simulink model "sampleModel2068_2_sub_sub"  (R2023a)
settings: Solver=VariableStepAuto  StartTime=0.0  StopTime=10.0  RelTol=1e-3
libraries: hdlsllib x2, simulink x2
settings Model: Creator=user1  LastModifiedBy=user1

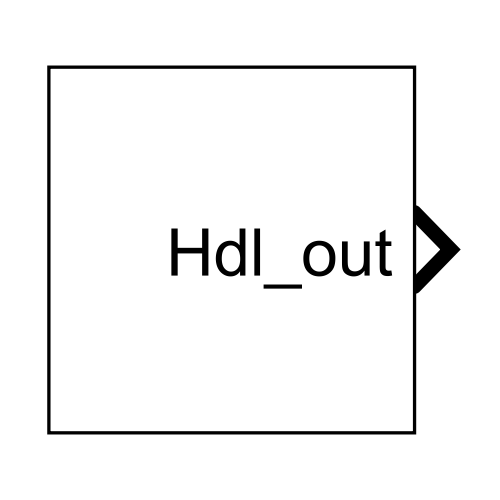
[thumbnail: Simulink's stored preview of the top-level diagram]
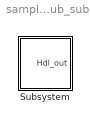
== system sampleModel2068_2_sub_sub ==
  Subsystem : Subsystem

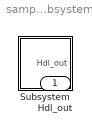
== system sampleModel2068_2_sub_sub/Subsystem ==
  Subsystem : Subsystem
  Hdl_out : Outport  OutDataTypeStr=uint8

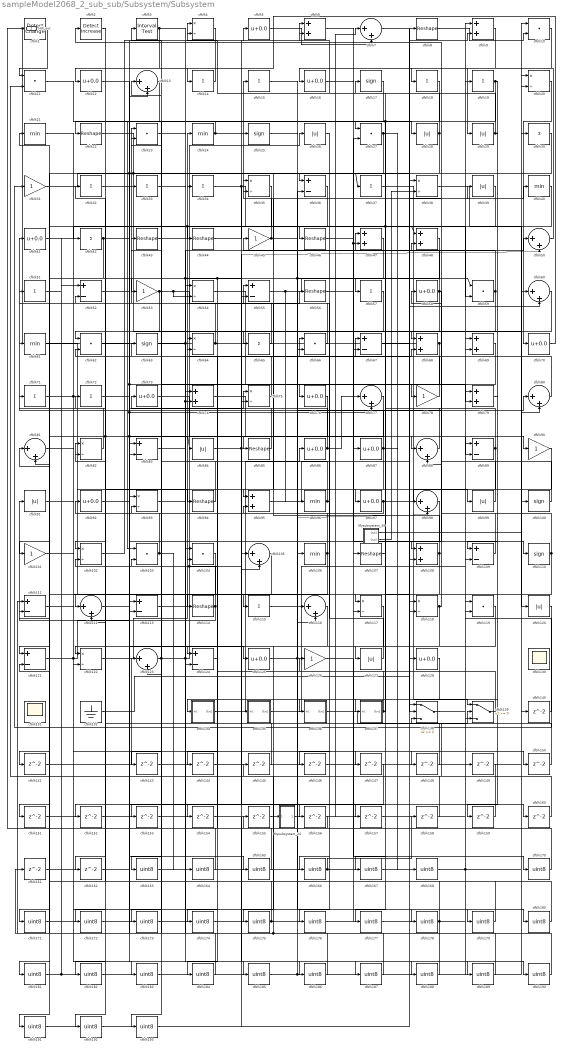
== system sampleModel2068_2_sub_sub/Subsystem/Subsystem ==
  Mysubsystem_24 : Subsystem  TreatAsAtomicUnit=on  RTWFcnName=Mysubsystem_24
      settings: RTWFcnNameOpts=User specified  RTWFileNameOpts=Use function name
  Mysubsystem_45 : Subsystem  TreatAsAtomicUnit=on  RTWFcnName=Mysubsystem_45
      settings: RTWFcnNameOpts=User specified  RTWFileNameOpts=Use function name
  cfblk1 : simulink/Logic and Bit Operations/Detect Change  vinit=0  OutDataTypeStr=uint8
      settings: LibrarySourceBlock=|
      | hdlsllib/Logic and Bit
      | Operations/Detect
      | Change
  cfblk{10..11,23,27,59,62,66,103..104,119} (10 alike) : DotProduct  OutDataTypeStr=uint8
  cfblk{17,25,63,100,110} (5 alike) : Signum
  cfblk{31,45,53,78,90,101,126} (7 alike) : Gain  OutDataTypeStr=uint8
  cfblk{4,20,35,38,54,64,75,82,93,102,117..118,122} (13 alike) : Product  Inputs=*/  OutDataTypeStr=uint8  RndMeth=Zero  SaturateOnIntegerOverflow=on
  cfblk{7,13,50,60,77,80..81,88,98,105,112,116,123} (13 alike) : Sum  Inputs=|++  OutDataTypeStr=uint8
  cfblk{21,24,40,61,96,106} (6 alike) : MinMax  OutDataTypeStr=uint8
  cfblk{8,22,43..44,46,56,85,94,107,114} (10 alike) : Reshape
  cfblk{6,9,47..48,68..69,74,79,95,108} (10 alike) : Sum  OutDataTypeStr=uint8
  cfblk{36,52,55,67,83,89,109,111,113,121,124} (11 alike) : Sum  Inputs=+-  OutDataTypeStr=uint8
  cfblk{14..15,18..19,30,32..34,37,42,51,57,65,71..72,115} (16 alike) : Sum  Inputs=+  OutDataTypeStr=uint8
  cfblk{5,12,16,41,58,70,73,76,86..87,92,97,125,128} (14 alike) : Bias  Bias=0.0  SaturateOnIntegerOverflow=off
  cfblk{26,28..29,39,84,91,99,120,127} (9 alike) : Abs  OutDataTypeStr=uint8  SaturateOnIntegerOverflow=off
  cfblk130 : Scope
      settings: Floating=on
  cfblk131 : Scope
      settings: Floating=on
  cfblk132 : Ground
  cfblk134 : Subsystem
      settings: LibrarySourceBlock=|
      | hdlsllib/Ports &
      | Subsystems/Subsystem
  cfblk135 : Subsystem
      settings: LibrarySourceBlock=|
      | hdlsllib/Ports &
      | Subsystems/Subsystem
  cfblk136 : Subsystem
      settings: LibrarySourceBlock=|
      | hdlsllib/Ports &
      | Subsystems/Subsystem
  cfblk137 : Subsystem
      settings: LibrarySourceBlock=|
      | hdlsllib/Ports &
      | Subsystems/Subsystem
  cfblk138 : Switch  OutDataTypeStr=uint8  SaturateOnIntegerOverflow=off  InputSameDT=off
  cfblk139 : Switch  OutDataTypeStr=uint8  SaturateOnIntegerOverflow=off  InputSameDT=off
  cfblk{140..141,143..162} (22 alike) : Delay  SampleTime=1
  cfblk{163..168,170..193} (30 alike) : DataTypeConversion  OutDataTypeStr=uint8  SaturateOnIntegerOverflow=off  RndMeth=Floor
  cfblk2 : simulink/Logic and Bit Operations/Detect Increase  vinit=0.0  OutDataTypeStr=uint8
      settings: LibrarySourceBlock=|
      | hdlsllib/Logic and Bit
      | Operations/Detect
      | Increase
  cfblk3 : hdlsllib/Logic and Bit Operations/Interval Test  IntervalClosedRight=on  uplimit=0.5  IntervalClosedLeft=on  lowlimit=-0.5  OutDataTypeStr=uint8
  Hdl_out : Outport  OutDataTypeStr=uint8
  wires:
  Mysubsystem_45/2(Out2) -> cfblk38/2
  Mysubsystem_45/1(Out1) -> cfblk10/1
  Mysubsystem_24/1(Out1) -> cfblk7/1
  cfblk83/1 -> Mysubsystem_24/1(In1)
  cfblk193/1 -> cfblk105/2
  cfblk60/1 -> cfblk193/1
  cfblk192/1 -> cfblk105/1
  cfblk147/1 -> cfblk192/1
  cfblk191/1 -> cfblk8/1
  cfblk105/1 -> cfblk191/1
  cfblk190/1 -> cfblk93/2
  cfblk154/1 -> cfblk190/1
  cfblk189/1 -> cfblk93/1
  cfblk188/1 -> cfblk155/1, cfblk74/1
  cfblk187/1 -> cfblk111/2
  cfblk92/1 -> cfblk187/1
  cfblk186/1 -> cfblk111/1
  cfblk91/1 -> cfblk186/1
  cfblk185/1 -> cfblk36/2, cfblk20/1
  cfblk184/1 -> cfblk21/1
  cfblk128/1 -> cfblk184/1
  cfblk183/1 -> cfblk20/2
  cfblk21/1 -> cfblk183/1
  cfblk182/1 -> cfblk30/1
  cfblk181/1 -> cfblk149/1, cfblk52/1
  cfblk180/1 -> cfblk81/2
  cfblk179/1 -> cfblk81/1
  cfblk178/1 -> cfblk161/1, cfblk38/1
  cfblk177/1 -> cfblk119/2
  cfblk176/1 -> cfblk119/1
  cfblk175/1 -> cfblk145/1, cfblk92/1
  cfblk174/1 -> cfblk116/2
  cfblk173/1 -> cfblk116/1
  cfblk36/1 -> cfblk173/1
  cfblk172/1 -> cfblk107/1
  cfblk116/1 -> cfblk172/1
  cfblk171/1 -> cfblk83/2
  cfblk170/1 -> cfblk83/1
  cfblk126/1 -> cfblk170/1
  cfblk168/1 -> cfblk69/2
  cfblk167/1 -> cfblk69/1
  cfblk166/1 -> cfblk139/3, cfblk80/2, cfblk158/1
  cfblk165/1 -> cfblk104/2
  cfblk62/1 -> cfblk165/1
  cfblk164/1 -> cfblk104/1
  cfblk163/1 -> cfblk140/1
  cfblk104/1 -> cfblk163/1
  cfblk162/1 -> cfblk82/2
  cfblk161/1 -> cfblk13/2
  cfblk160/1 -> cfblk9/1
  cfblk15/1 -> cfblk160/1
  cfblk159/1 -> cfblk138/3
  cfblk158/1 -> cfblk121/2
  cfblk157/1 -> cfblk108/2
  cfblk156/1 -> cfblk1/1
  cfblk155/1 -> cfblk109/2
  cfblk153/1 -> cfblk117/2
  cfblk68/1 -> cfblk153/1, Hdl_out/1
  cfblk152/1 -> cfblk66/2
  cfblk151/1 -> cfblk27/2
  cfblk150/1 -> cfblk113/1
  cfblk101/1 -> cfblk150/1
  cfblk149/1 -> cfblk11/2
  cfblk148/1 -> cfblk102/2
  cfblk146/1 -> cfblk67/2
  cfblk145/1 -> cfblk103/2
  cfblk144/1 -> cfblk89/1
  cfblk124/1 -> cfblk144/1
  cfblk143/1 -> cfblk60/1
  cfblk17/1 -> cfblk143/1
  cfblk141/1 -> cfblk123/1
  cfblk39/1 -> cfblk141/1
  cfblk140/1 -> cfblk79/1
  cfblk32/1 -> cfblk79/2, cfblk118/2
  cfblk127/1 -> cfblk51/1
  cfblk79/1 -> cfblk109/1
  cfblk2/1 -> cfblk102/1
  cfblk35/1 -> cfblk122/2
  cfblk3/1 -> cfblk55/2, cfblk148/1, cfblk122/1
  cfblk95/1 -> cfblk39/1
  cfblk132/1 -> cfblk118/1
  cfblk1/1 -> cfblk11/1
  cfblk106/1 -> cfblk52/2, cfblk154/1
  cfblk117/1 -> cfblk123/2
  cfblk53/1 -> cfblk56/1, cfblk54/2, cfblk152/1
  cfblk110/1 -> cfblk35/1, cfblk167/1
  cfblk11/1 -> cfblk28/1
  cfblk46/1 -> cfblk89/2
  cfblk108/1 -> cfblk55/1, cfblk138/2
  cfblk25/1 -> cfblk59/1, cfblk179/1
  cfblk67/1 -> cfblk9/2
  cfblk28/1 -> cfblk65/1, cfblk6/2
  cfblk24/1 -> cfblk22/1, cfblk6/1
  cfblk18/1 -> cfblk27/1
  cfblk72/1 -> cfblk84/1, cfblk156/1
  cfblk71/1 -> cfblk94/1, cfblk114/1
  cfblk9/1 -> cfblk18/1
  cfblk52/1 -> cfblk4/1
  cfblk93/1 -> cfblk188/1
  cfblk107/1 -> cfblk137/1(In1)
  cfblk63/1 -> cfblk68/1, cfblk189/1
  cfblk65/1 -> cfblk32/1
  cfblk56/1 -> cfblk48/2
  cfblk47/1 -> cfblk136/1(In1)
  cfblk115/1 -> cfblk80/1
  cfblk48/1 -> cfblk151/1, cfblk174/1
  cfblk103/1 -> cfblk82/1, cfblk164/1
  cfblk99/1 -> cfblk71/1
  cfblk84/1 -> cfblk50/2, cfblk157/1
  cfblk7/1 -> cfblk60/2
  cfblk5/1 -> cfblk7/2
  cfblk100/1 -> cfblk58/1
  cfblk4/1 -> cfblk112/2
  cfblk54/1 -> cfblk128/1
  cfblk23/1 -> cfblk54/1
  cfblk96/1 -> cfblk43/1, cfblk146/1
  cfblk122/1 -> cfblk64/1
  cfblk81/1 -> cfblk178/1
  cfblk44/1 -> cfblk25/1
  cfblk8/1 -> cfblk10/2
  cfblk58/1 -> cfblk74/2, cfblk124/2, cfblk108/1, cfblk35/2
  cfblk30/1 -> cfblk181/1
  cfblk41/1 -> cfblk48/1, cfblk44/1
  cfblk12/1 -> cfblk37/1, cfblk115/1
  cfblk94/1 -> cfblk73/1
  cfblk78/1 -> cfblk66/1
  cfblk82/1 -> cfblk61/1
  cfblk98/1 -> cfblk113/2
  cfblk38/1 -> cfblk120/1
  cfblk125/1 -> cfblk98/2, cfblk147/1
  cfblk120/1 -> cfblk31/1
  cfblk97/1 -> cfblk95/2, cfblk99/1
  cfblk69/1 -> cfblk166/1
  cfblk121/1 -> cfblk33/1, cfblk180/1
  cfblk19/1 -> cfblk53/1, cfblk97/1, cfblk159/1
  cfblk86/1 -> cfblk13/1, cfblk77/1
  cfblk14/1 -> cfblk12/1
  cfblk64/1 -> cfblk23/1, cfblk124/1
  cfblk6/1 -> cfblk87/1
  cfblk57/1 -> cfblk95/1
  cfblk139/1 -> cfblk126/1
  cfblk42/1 -> cfblk125/1, cfblk77/2, cfblk171/1
  cfblk33/1 -> cfblk78/1
  cfblk16/1 -> cfblk47/2, cfblk110/1
  cfblk135/1(Out1) -> cfblk19/1
  cfblk118/1 -> cfblk88/2, cfblk177/1
  cfblk112/1 -> cfblk75/1
  cfblk109/1 -> cfblk2/1
  cfblk76/1 -> cfblk101/1, cfblk182/1
  cfblk22/1 -> cfblk100/1, cfblk138/1
  cfblk90/1 -> cfblk112/1
  cfblk85/1 -> cfblk34/1
  cfblk138/1 -> cfblk40/1
  cfblk43/1 -> cfblk46/1
  cfblk73/1 -> cfblk88/1
  cfblk40/1 -> cfblk127/1, cfblk75/2
  cfblk137/1(Out1) -> cfblk17/1, cfblk64/2
  cfblk119/1 -> cfblk175/1
  cfblk20/1 -> cfblk70/1
  cfblk136/1(Out1) -> cfblk139/2
  cfblk27/1 -> cfblk121/1, cfblk98/1
  cfblk37/1 -> cfblk139/1
  cfblk123/1 -> cfblk67/1, cfblk68/2, cfblk50/1, cfblk23/2
  cfblk113/1 -> cfblk26/1
  cfblk26/1 -> cfblk76/1
  cfblk80/1 -> cfblk47/1
  cfblk45/1 -> cfblk15/1, cfblk90/1
  cfblk61/1 -> cfblk117/1
  cfblk87/1 -> cfblk41/1, cfblk162/1, cfblk168/1
  cfblk74/1 -> cfblk106/1
  cfblk77/1 -> cfblk85/1
  cfblk55/1 -> cfblk57/1, cfblk96/1
  cfblk34/1 -> cfblk135/1(In1), cfblk59/2
  cfblk59/1 -> cfblk45/1, cfblk62/1
  cfblk31/1 -> cfblk36/1
  cfblk134/1(Out1) -> cfblk86/1
  cfblk75/1 -> cfblk3/1
  cfblk66/1 -> cfblk24/1
  cfblk51/1 -> cfblk42/1
  cfblk70/1 -> cfblk14/1
  cfblk10/1 -> cfblk29/1
  cfblk29/1 -> cfblk134/1(In1), cfblk4/2
  cfblk50/1 -> cfblk16/1
  cfblk114/1 -> cfblk91/1, cfblk72/1
  cfblk111/1 -> cfblk185/1
  cfblk102/1 -> cfblk5/1
  cfblk13/1 -> cfblk103/1
  cfblk89/1 -> cfblk62/2, cfblk176/1
  cfblk88/1 -> cfblk63/1

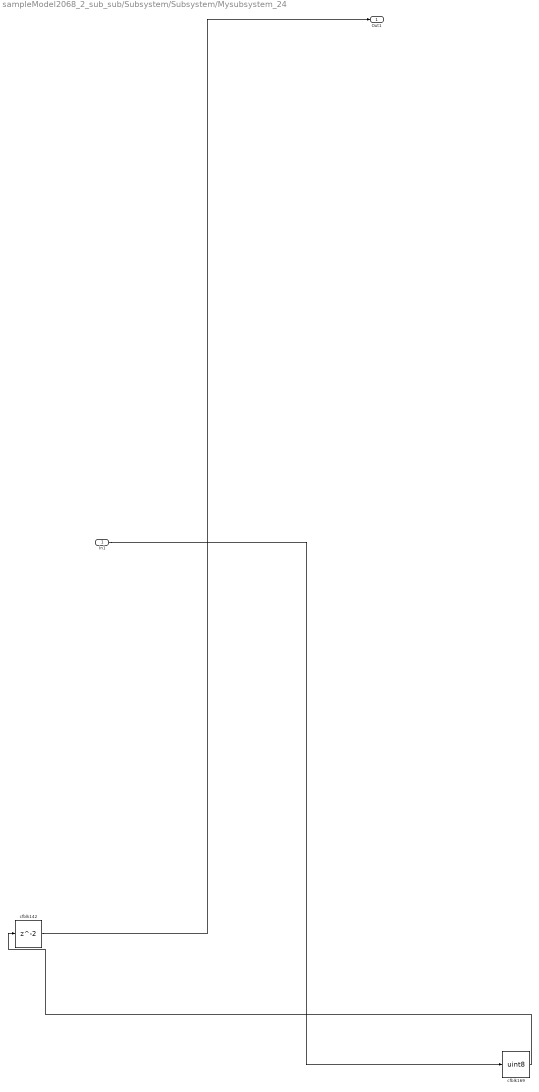
== system sampleModel2068_2_sub_sub/Subsystem/Subsystem/Mysubsystem_24 ==
  In1 : Inport
  cfblk142 : Delay  SampleTime=1
  cfblk169 : DataTypeConversion  OutDataTypeStr=uint8  SaturateOnIntegerOverflow=off  RndMeth=Floor
  Out1 : Outport
  wires:
  cfblk142/1 -> Out1/1
  cfblk169/1 -> cfblk142/1
  In1/1 -> cfblk169/1

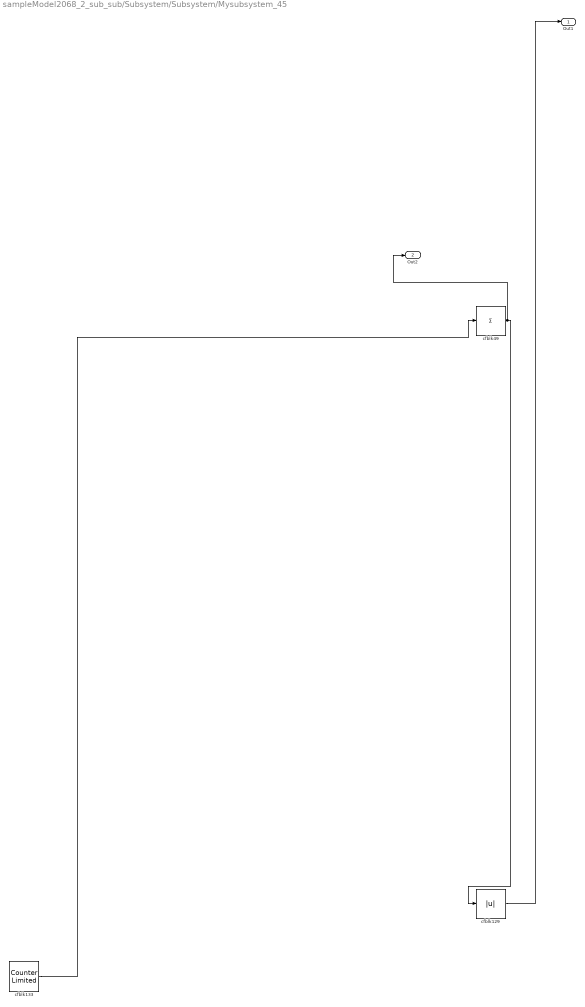
== system sampleModel2068_2_sub_sub/Subsystem/Subsystem/Mysubsystem_45 ==
  cfblk129 : Abs  SaturateOnIntegerOverflow=off
  cfblk133 : hdlsllib/Sources/Counter Limited  uplimit=7  tsamp=-1
  cfblk49 : Sum  Inputs=+
  Out1 : Outport
  Out2 : Outport  Port=2
  wires:
  cfblk49/1 -> Out2/1, cfblk129/1
  cfblk133/1 -> cfblk49/1
  cfblk129/1 -> Out1/1

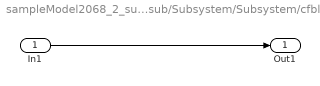
== system sampleModel2068_2_sub_sub/Subsystem/Subsystem/cfblk134 ==
  In1 : Inport
  Out1 : Outport
  wires:
  In1/1 -> Out1/1

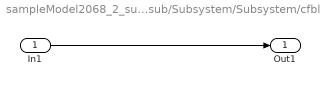
== system sampleModel2068_2_sub_sub/Subsystem/Subsystem/cfblk135 ==
  In1 : Inport
  Out1 : Outport
  wires:
  In1/1 -> Out1/1

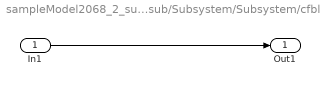
== system sampleModel2068_2_sub_sub/Subsystem/Subsystem/cfblk136 ==
  In1 : Inport
  Out1 : Outport
  wires:
  In1/1 -> Out1/1

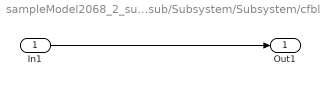
== system sampleModel2068_2_sub_sub/Subsystem/Subsystem/cfblk137 ==
  In1 : Inport
  Out1 : Outport
  wires:
  In1/1 -> Out1/1
